simulink library "vmc"  (R2021b)
settings: Solver=VariableStepAuto  StartTime=0.0  StopTime=10.0  RelTol=1e-3
undefined symbols (not defined in the file): AVMC_ACCDeltaTqGradeGn_X_deg, AVMC_ACCDeltaTqIGain4OVRD_X_kph, AVMC_ACCDeltaTqIGain4OVRD_Y_mps2, AVMC_ACCDeltaTqIGain_X_kph, AVMC_ACCDeltaTqIGain_Y_mps2, AVMC_ACCDeltaTqPGain_X_kph, AVMC_ACCDeltaTqPGain_Y_kph, AVMC_ACCGradeofst_X_G, AVMC_ACCGradeofst_Y_pct, AVMC_ACCLoSpdTqLoLim4JP_X_kph, AVMC_ACCLoSpdTqLoLim4JP_Y_deg, AVMC_ACCLoSpdTqLowerLim_X_kph, AVMC_ACCLoSpdTqLowerLim_Y_deg, AVMC_ACCReqAccelGain_X_mps2, AVMC_ACCReqAccelGain_Y_enum, AVMC_ADSPosGFBDeltaTq_X_kph, AVMC_ADSPosGFBDeltaTq_Y_mps2, AVMC_AggressJerkPCT4AT_X_kph, AVMC_AggressJerkPCT_X_kph, AVMC_AggressLimitPCT4AT_X_kph, AVMC_AggressLimitPCT_X_kph, AVMC_DECGradeofst_X_G, AVMC_DECGradeofst_Y_pct, AVMC_DISCDeltaTqIGain_X_kph, AVMC_DISCDeltaTqIGain_Y_mps2, AVMC_DISCDeltaTqPGain_X_kph, AVMC_DISCDeltaTqPGain_Y_kph, AVMC_EPSForceSelect_X_enum, AVMC_EPSForceSelect_Y_enum, AVMC_EPSForceSelectD21_X_enum, AVMC_EPSForceSelectD21_Y_enum, AVMC_ESCRegenOut_X_kph, AVMC_ESCRegenOut_Y_Deg, AVMC_ESCRegenOutEnSpd_X_Deg, AVMC_EstPitchSlopeTs_X_kph, AVMC_GradeCompFlt_X_kph, AVMC_GyroYBandLo_X_Gps, AVMC_HoldResTq_X_kph, AVMC_ISOAccLimit_X_mps, AVMC_ISODecLimit_X_mps, AVMC_ISOJerk_X_mps, AVMC_LatESCRegenOut_X_kph, AVMC_LatESCRegenOut_Y_Deg, AVMC_LongAccDeadZone_X_kph, AVMC_LongAccFiltTsforP2_X_Gps, AVMC_MCPresBaseTq_X_bar, AVMC_MSAPedalOvrd_X_kph, AVMC_MSASpdBand_X_kph, AVMC_MSATqDownEndTq_X_kph, AVMC_MSATqDownTime_X_kph, AVMC_NegZCHoldTq_X_kph, AVMC_OPDDisSlideRate_X_Deg, AVMC_OVRD2ActSR2FCMCMD_X_mps2, AVMC_PedalTqRWhlRatio_X_Nm, AVMC_PedalTqRWhlRatio_Y_gps, AVMC_PedalTqRWhlSlipGain_X_rat, AVMC_PedalTqRWhlSlipGain_Y_kph, AVMC_PedalTqRWhSTRGGain_X_deg, AVMC_PedalTqRWhSTRGGain_Y_kph, AVMC_PosZCHoldTq_X_kph ... (+593)
libraries: hcu_lib x143, simulink x96, tqr x4, $bdroot x1, simulink_extras x1
(part 16 of 17)

== system vmc/VMC/VMC/Slide Rate  Calculation/4Wheel Calculation/RR Wheel ==
  VVMC_4WheelLongAcc_Gps : Inport
  task_time_s : Inport  Port=2
  VINP_RRRawWhlSpeed_kph : Inport  Port=3
  VTQD_GearActualPosn_enum : Inport  Port=4
  AND4 : Logic  Inputs=3  AllPortsSameDT=off  OutDataTypeStr=boolean
  Abs3 : Abs
  Add : Sum
  Add{3,8,15..16} (4 alike) : Sum  Inputs=+-
  Constant1 : Constant  Value=GRAVITY_G
  Constant11 : Constant  Value=KPH2MPS
  Constant14 : Constant  Value=ONE_PERCENT
  Constant15 : Constant  Value=KVMC_RawWhlSpeedDeadZone_kph
  Constant16 : Constant  Value=ZERO_FLOAT
  Constant17 : Constant  Value=KVMC_RawWhlSpeedDeadZone_kph
  Constant18 : Constant  Value=ONE_FLOAT
  Constant2 : Constant  Value=MPS2KPH
  Constant33 : Constant  Value=KPH2MPS
  Constant34 : Constant  Value=GRAVITY_G
  Constant35 : Constant  Value=KVMC_WhlSpdCalAccTs_c
  Constant42 : Constant  Value=KVMC_WheelSkidAccDev_Gps
  Constant43 : Constant  Value=KVMC_SkidRecVehSpdDev_kph
  Constant44 : Constant  Value=KPH2MPS
  Constant46 : Constant  Value=ENUM_GEARACTUALPOSN_D
  Constant47 : Constant  Value=ENUM_GEARACTUALPOSN_R
  Constant48 : Constant  Value=KVMC_PreVehSpdCalSW_flg
  Constant49 : Constant  Value=KVMC_RRWhlSkidReset_flg
  Constant5 : Constant  Value=KVMC_4WheelEnSkidDetSpd_kph
  Delay{,4..5,12..13,17} (6 alike) : Delay  DelayLength=1
  Divide3 : Product  Inputs=*//
  Divide7 : Product  Inputs=**//
  Equal : RelationalOperator  Operator===  OutDataTypeStr=boolean  RndMeth=Simplest
  Equal1 : RelationalOperator  Operator===  OutDataTypeStr=boolean  RndMeth=Simplest
  FirstOrderFilter3 : hcu_lib/Basic_Blocks/FirstOrderFilter
  OR : Logic  Operator=OR  AllPortsSameDT=off  OutDataTypeStr=boolean
  OR1 : Logic  Operator=OR  AllPortsSameDT=off  OutDataTypeStr=boolean
  OR2 : Logic  Operator=OR  AllPortsSameDT=off  OutDataTypeStr=boolean
  Product : Product
  Product1 : Product  Inputs=3
  Product2 : Product
  Product3 : Product
  Relational Operator14 : RelationalOperator  Operator=>  OutDataTypeStr=boolean  RndMeth=Simplest
  Relational Operator{2,5..6,15} (4 alike) : RelationalOperator  Operator=<=  OutDataTypeStr=boolean  RndMeth=Simplest
  SR_Latch3 : hcu_lib/Basic_Blocks/SR_Latch
  Saturation : Saturate  UpperLimit=KVMC_PredVehSpdLimit_mps  LowerLimit=ZERO_FLOAT
  Switch{,5..6,10} (4 alike) : Switch  Criteria=u2 > Threshold
  VVMC_RRPreVehSpd_kph : Outport
  VVMC_RRWhlSkid_flg : Outport  Port=2
  VVMC_RR4WhlSpdSlideRate_pct : Outport  Port=3
  wires:
  OR2/1 -> SR_Latch3/2  "VVMC_RRWhlSkidReset_flg"
  AND4/1 -> OR2/2
  Relational Operator2/1 -> OR2/1
  [VINP_RRRawWhlSpeed_kph] -> Relational Operator2/1
  Constant5/1 -> Relational Operator2/2
  [VVMC_RR4WhlSpdSlideRate_pct] -> VVMC_RR4WhlSpdSlideRate_pct/1
  [VVMC_RRWhlSkid_flg] -> VVMC_RRWhlSkid_flg/1
  [VVMC_RRPreVehSpd_kph] -> VVMC_RRPreVehSpd_kph/1
  VINP_RRRawWhlSpeed_kph/1 -> [VINP_RRRawWhlSpeed_kph]
  task_time_s/1 -> [task_time_s]
  VTQD_GearActualPosn_enum/1 -> [VTQD_GearActualPosn_enum]
  VVMC_4WheelLongAcc_Gps/1 -> [VVMC_4WheelLongAcc_Gps]
  [VVMC_RRPreVehSpd_kph] -> Switch5/3
  [VVMC_RRPreVehSpd_kph] -> Relational Operator5/1
  [VVMC_RRPreVehSpd_kph] -> Add3/2
  [VVMC_RRPreVehSpd_kph] -> Delay12/1
  [VINP_RRRawWhlSpeed_kph] -> Delay13/1
  [VINP_RRRawWhlSpeed_kph] -> Delay/1
  [VVMC_RRWhlSkid_flg] -> OR1/1
  OR/1 -> Switch10/2
  Product/1 -> Switch/3
  Delay5/1 -> Product3/1
  Saturation/1 -> Add/2
  Product1/1 -> Add/1  "VVMC_RRDeltaVehSpd_mps"
  Constant46/1 -> Equal/2
  OR1/1 -> Switch/2
  Constant2/1 -> Product2/2
  Constant48/1 -> OR1/2
  [VTQD_GearActualPosn_enum] -> Equal1/1
  Equal1/1 -> OR/2
  Constant47/1 -> Equal1/2
  Delay/1 -> Product/1
  [VVMC_RRPreVehSpd_kph] -> Delay5/1
  Switch/1 -> Saturation/1  "VVMC_RRLastPreVehSpd_mps"
  [task_time_s] -> Product1/3
  Constant44/1 -> Product3/2
  Constant11/1 -> Product/2
  [VVMC_4WheelLongAcc_Gps] -> Product1/1
  Product2/1 -> Switch10/1
  Equal/1 -> OR/1
  Add/1 -> Product2/1  "VVMC_RRCalPreVehSpd_mps"
  [VTQD_GearActualPosn_enum] -> Equal/1
  [VINP_RRRawWhlSpeed_kph] -> Switch10/3
  Switch10/1 -> [VVMC_RRPreVehSpd_kph]  "VVMC_RRPreVehSpd_kph"
  Constant1/1 -> Product1/2
  Product3/1 -> Switch/1
  Add3/1 -> Divide3/1
  [VINP_RRRawWhlSpeed_kph] -> Add3/1
  Constant17/1 -> Relational Operator5/2
  Constant16/1 -> Switch6/1
  Constant15/1 -> Relational Operator6/2
  Relational Operator5/1 -> Switch5/2
  [VINP_RRRawWhlSpeed_kph] -> Relational Operator6/1
  Relational Operator6/1 -> Switch6/2
  Constant18/1 -> Switch5/1
  Switch6/1 -> [VVMC_RR4WhlSpdSlideRate_pct]  "VVMC_RR4WhlSpdSlideRate_pct"
  Divide3/1 -> Switch6/3  "VVMC_RRCal4WhlSpdSlideRate_pct"
  Switch5/1 -> Divide3/3
  Constant14/1 -> Divide3/2
  Constant35/1 -> FirstOrderFilter3/3
  [VVMC_RRWhlCalAcc_Gps] -> Add16/1
  SR_Latch3/1 -> [VVMC_RRWhlSkid_flg]  "VVMC_RRWhlSkid_flg"
  Abs3/1 -> Relational Operator15/1
  Constant34/1 -> Divide7/4
  Constant33/1 -> Divide7/2
  Delay13/1 -> Add15/2
  Constant43/1 -> Relational Operator15/2
  Delay12/1 -> Add15/1
  Add16/1 -> Relational Operator14/1
  [VVMC_RRWhlSkid_flg] -> Delay17/1
  Delay17/1 -> AND4/2
  Delay4/1 -> Add8/2
  Relational Operator15/1 -> AND4/1
  Divide7/1 -> FirstOrderFilter3/1
  FirstOrderFilter3/1 -> [VVMC_RRWhlCalAcc_Gps]  "VVMC_RRWhlCalAcc_Gps"
  Constant42/1 -> Relational Operator14/2
  [VINP_RRRawWhlSpeed_kph] -> Delay4/1
  [task_time_s] -> FirstOrderFilter3/2
  [VVMC_4WheelLongAcc_Gps] -> Add16/2
  Relational Operator14/1 -> SR_Latch3/1
  Add15/1 -> Abs3/1
  [task_time_s] -> Divide7/3
  Add8/1 -> Divide7/1
  Constant49/1 -> AND4/3
  [VINP_RRRawWhlSpeed_kph] -> Add8/1

== stateflow chart vmc/VMC/VMC/IMU/IMU sensing result /RollingAverage3 ==
  state RollingAverage
    (default) -> (junction 2) : {VVMC_RollAveCount_enum = ONE_INT}
    RollingAverage -> (junction 2)
    (junction 2) -> (junction 3) : {VVMC_RollAve_raw32 = ZERO_FLOAT}
    (junction 3) -> (junction 100) [order 1] : [VVMC_RollAveCount_enum < KVMC_RollAveLevel_enum]
    (junction 3) -> (junction 37) [order 2]
    (junction 100) -> (junction 5) : {% Memory
        |  VVMC_Memory_raw32[VVMC_RollAveCount_enum] = VINP_INPData_raw32;
        |
        |  % Memory Shift Counter
        |  VVMC_ShiftCount_enum = ONE_INT}
    (junction 5) -> (junction 7) [order 2]
    (junction 5) -> (junction 6) [order 1] : [VVMC_ShiftCount_enum <= VVMC_RollAveCount_enum]
    (junction 7) -> (junction 8) : {% Rolling Average
        |  VVMC_RollAve_raw32 = VVMC_RollAve_raw32 / VVMC_RollAveCount_enum;
        |
        |  % Rolling Average Counter
        |  VVMC_RollAveCount_enum++}
    (junction 35) -> (junction 5) : {VVMC_ShiftCount_enum++}
    (junction 6) -> (junction 36) : {% Rolling Average Sum
        |  VVMC_RollAve_raw32 = VVMC_RollAve_raw32 + VVMC_Memory_raw32[VVMC_ShiftCount_enum];
        |  }
    (junction 36) -> (junction 35)
    (junction 37) -> (junction 76) [order 1] : [VVMC_RollAveCount_enum == KVMC_RollAveLevel_enum]
    (junction 76) -> (junction 47)
    (junction 37) -> (junction 60) [order 2]
    (junction 78) -> (junction 76)
    (junction 47) -> (junction 30) : {% Memory
        |  VVMC_Memory_raw32[VVMC_RollAveCount_enum] = VINP_INPData_raw32;
        |
        |  % Memory Shift Counter
        |  VVMC_ShiftCount_enum = ONE_INT;
        | }
    (junction 60) -> (junction 62) [order 1] : [VVMC_RollAveCount_enum > KVMC_RollAveLevel_enum]
    (junction 60) -> (junction 39) [order 2]
    (junction 62) -> (junction 66) : {VVMC_MemoryShiftCount_enum = ONE_INT}
    (junction 30) -> (junction 48) [order 2]
    (junction 30) -> (junction 22) [order 1] : [VVMC_ShiftCount_enum <= VVMC_RollAveCount_enum]
    (junction 48) -> (junction 45) : {% Rolling Average
        |  VVMC_RollAve_raw32 = VVMC_RollAve_raw32 / VVMC_RollAveCount_enum;
        |
        |  % Memory Shift Counter
        |  VVMC_ShiftCount_enum = ONE_INT}
    (junction 14) -> (junction 30) : {VVMC_ShiftCount_enum++}
    (junction 22) -> (junction 25) : {% Rolling Average Sum
        |  VVMC_RollAve_raw32 = VVMC_RollAve_raw32 + VVMC_Memory_raw32[VVMC_ShiftCount_enum]}
    (junction 66) -> (junction 82) [order 2]
    (junction 66) -> (junction 69) [order 1] : [VVMC_MemoryShiftCount_enum < VVMC_RollAveCount_enum]
    (junction 82) -> (junction 80) : {VVMC_RollAveCount_enum = KVMC_RollAveLevel_enum}
    (junction 73) -> (junction 66) : {VVMC_MemoryShiftCount_enum++}
    (junction 69) -> (junction 71) : {VVMC_Memory_raw32[VVMC_MemoryShiftCount_enum] =...
        |  VVMC_Memory_raw32[VVMC_RollAveCount_enum - KVMC_RollAveLevel_enum + VVMC_MemoryShiftCount_enum]}
    (junction 25) -> (junction 14)
    (junction 71) -> (junction 73)
    (junction 80) -> (junction 78)
    (junction 45) -> (junction 39) [order 2]
    (junction 45) -> (junction 15) [order 1] : [VVMC_ShiftCount_enum < VVMC_RollAveCount_enum]
    (junction 41) -> (junction 45) : { VVMC_ShiftCount_enum++}
    (junction 15) -> (junction 38) : {% Gy Memory Shift
        |  VVMC_Memory_raw32[VVMC_ShiftCount_enum] = VVMC_Memory_raw32[VVMC_ShiftCount_enum + ONE_INT]}
    (junction 38) -> (junction 41)
  data: KVMC_RollAveLevel_enum input uint8; VVMC_ShiftCount_enum local uint8; VVMC_RollAveCount_enum local uint8; VVMC_Memory_raw32 local single size=256; ZERO_FLOAT input single; ONE_INT input uint8; VVMC_RollAve_raw32 output single; VINP_INPData_raw32 input single; VVMC_MemoryShiftCount_enum local uint8

== stateflow chart vmc/VMC/VMC/IMU/IMU sensing result /RollingAverage4 ==
  state RollingAverage
    (default) -> (junction 2) : {VVMC_RollAveCount_enum = ONE_INT}
    RollingAverage -> (junction 2)
    (junction 2) -> (junction 3) : {VVMC_RollAve_raw32 = ZERO_FLOAT}
    (junction 3) -> (junction 100) [order 1] : [VVMC_RollAveCount_enum < KVMC_RollAveLevel_enum]
    (junction 3) -> (junction 37) [order 2]
    (junction 100) -> (junction 5) : {% Memory
        |  VVMC_Memory_raw32[VVMC_RollAveCount_enum] = VINP_INPData_raw32;
        |
        |  % Memory Shift Counter
        |  VVMC_ShiftCount_enum = ONE_INT}
    (junction 5) -> (junction 7) [order 2]
    (junction 5) -> (junction 6) [order 1] : [VVMC_ShiftCount_enum <= VVMC_RollAveCount_enum]
    (junction 7) -> (junction 8) : {% Rolling Average
        |  VVMC_RollAve_raw32 = VVMC_RollAve_raw32 / VVMC_RollAveCount_enum;
        |
        |  % Rolling Average Counter
        |  VVMC_RollAveCount_enum++}
    (junction 35) -> (junction 5) : {VVMC_ShiftCount_enum++}
    (junction 6) -> (junction 36) : {% Rolling Average Sum
        |  VVMC_RollAve_raw32 = VVMC_RollAve_raw32 + VVMC_Memory_raw32[VVMC_ShiftCount_enum];
        |  }
    (junction 36) -> (junction 35)
    (junction 37) -> (junction 76) [order 1] : [VVMC_RollAveCount_enum == KVMC_RollAveLevel_enum]
    (junction 76) -> (junction 47)
    (junction 37) -> (junction 60) [order 2]
    (junction 78) -> (junction 76)
    (junction 47) -> (junction 30) : {% Memory
        |  VVMC_Memory_raw32[VVMC_RollAveCount_enum] = VINP_INPData_raw32;
        |
        |  % Memory Shift Counter
        |  VVMC_ShiftCount_enum = ONE_INT;
        | }
    (junction 60) -> (junction 62) [order 1] : [VVMC_RollAveCount_enum > KVMC_RollAveLevel_enum]
    (junction 60) -> (junction 39) [order 2]
    (junction 62) -> (junction 66) : {VVMC_MemoryShiftCount_enum = ONE_INT}
    (junction 30) -> (junction 48) [order 2]
    (junction 30) -> (junction 22) [order 1] : [VVMC_ShiftCount_enum <= VVMC_RollAveCount_enum]
    (junction 48) -> (junction 45) : {% Rolling Average
        |  VVMC_RollAve_raw32 = VVMC_RollAve_raw32 / VVMC_RollAveCount_enum;
        |
        |  % Memory Shift Counter
        |  VVMC_ShiftCount_enum = ONE_INT}
    (junction 14) -> (junction 30) : {VVMC_ShiftCount_enum++}
    (junction 22) -> (junction 25) : {% Rolling Average Sum
        |  VVMC_RollAve_raw32 = VVMC_RollAve_raw32 + VVMC_Memory_raw32[VVMC_ShiftCount_enum]}
    (junction 66) -> (junction 82) [order 2]
    (junction 66) -> (junction 69) [order 1] : [VVMC_MemoryShiftCount_enum < VVMC_RollAveCount_enum]
    (junction 82) -> (junction 80) : {VVMC_RollAveCount_enum = KVMC_RollAveLevel_enum}
    (junction 73) -> (junction 66) : {VVMC_MemoryShiftCount_enum++}
    (junction 69) -> (junction 71) : {VVMC_Memory_raw32[VVMC_MemoryShiftCount_enum] =...
        |  VVMC_Memory_raw32[VVMC_RollAveCount_enum - KVMC_RollAveLevel_enum + VVMC_MemoryShiftCount_enum]}
    (junction 25) -> (junction 14)
    (junction 71) -> (junction 73)
    (junction 80) -> (junction 78)
    (junction 45) -> (junction 39) [order 2]
    (junction 45) -> (junction 15) [order 1] : [VVMC_ShiftCount_enum < VVMC_RollAveCount_enum]
    (junction 41) -> (junction 45) : { VVMC_ShiftCount_enum++}
    (junction 15) -> (junction 38) : {% Gy Memory Shift
        |  VVMC_Memory_raw32[VVMC_ShiftCount_enum] = VVMC_Memory_raw32[VVMC_ShiftCount_enum + ONE_INT]}
    (junction 38) -> (junction 41)
  data: KVMC_RollAveLevel_enum input uint8; VVMC_ShiftCount_enum local uint8; VVMC_RollAveCount_enum local uint8; VVMC_Memory_raw32 local single size=256; ZERO_FLOAT input single; ONE_INT input uint8; VVMC_RollAve_raw32 output single; VINP_INPData_raw32 input single; VVMC_MemoryShiftCount_enum local uint8

== stateflow chart vmc/VMC/VMC/IMU/IMU sensing result /RollingAverage5 ==
  state RollingAverage
    (default) -> (junction 2) : {VVMC_RollAveCount_enum = ONE_INT}
    RollingAverage -> (junction 2)
    (junction 2) -> (junction 3) : {VVMC_RollAve_raw32 = ZERO_FLOAT}
    (junction 3) -> (junction 100) [order 1] : [VVMC_RollAveCount_enum < KVMC_RollAveLevel_enum]
    (junction 3) -> (junction 37) [order 2]
    (junction 100) -> (junction 5) : {% Memory
        |  VVMC_Memory_raw32[VVMC_RollAveCount_enum] = VINP_INPData_raw32;
        |
        |  % Memory Shift Counter
        |  VVMC_ShiftCount_enum = ONE_INT}
    (junction 5) -> (junction 7) [order 2]
    (junction 5) -> (junction 6) [order 1] : [VVMC_ShiftCount_enum <= VVMC_RollAveCount_enum]
    (junction 7) -> (junction 8) : {% Rolling Average
        |  VVMC_RollAve_raw32 = VVMC_RollAve_raw32 / VVMC_RollAveCount_enum;
        |
        |  % Rolling Average Counter
        |  VVMC_RollAveCount_enum++}
    (junction 35) -> (junction 5) : {VVMC_ShiftCount_enum++}
    (junction 6) -> (junction 36) : {% Rolling Average Sum
        |  VVMC_RollAve_raw32 = VVMC_RollAve_raw32 + VVMC_Memory_raw32[VVMC_ShiftCount_enum];
        |  }
    (junction 36) -> (junction 35)
    (junction 37) -> (junction 76) [order 1] : [VVMC_RollAveCount_enum == KVMC_RollAveLevel_enum]
    (junction 76) -> (junction 47)
    (junction 37) -> (junction 60) [order 2]
    (junction 78) -> (junction 76)
    (junction 47) -> (junction 30) : {% Memory
        |  VVMC_Memory_raw32[VVMC_RollAveCount_enum] = VINP_INPData_raw32;
        |
        |  % Memory Shift Counter
        |  VVMC_ShiftCount_enum = ONE_INT;
        | }
    (junction 60) -> (junction 62) [order 1] : [VVMC_RollAveCount_enum > KVMC_RollAveLevel_enum]
    (junction 60) -> (junction 39) [order 2]
    (junction 62) -> (junction 66) : {VVMC_MemoryShiftCount_enum = ONE_INT}
    (junction 30) -> (junction 48) [order 2]
    (junction 30) -> (junction 22) [order 1] : [VVMC_ShiftCount_enum <= VVMC_RollAveCount_enum]
    (junction 48) -> (junction 45) : {% Rolling Average
        |  VVMC_RollAve_raw32 = VVMC_RollAve_raw32 / VVMC_RollAveCount_enum;
        |
        |  % Memory Shift Counter
        |  VVMC_ShiftCount_enum = ONE_INT}
    (junction 14) -> (junction 30) : {VVMC_ShiftCount_enum++}
    (junction 22) -> (junction 25) : {% Rolling Average Sum
        |  VVMC_RollAve_raw32 = VVMC_RollAve_raw32 + VVMC_Memory_raw32[VVMC_ShiftCount_enum]}
    (junction 66) -> (junction 82) [order 2]
    (junction 66) -> (junction 69) [order 1] : [VVMC_MemoryShiftCount_enum < VVMC_RollAveCount_enum]
    (junction 82) -> (junction 80) : {VVMC_RollAveCount_enum = KVMC_RollAveLevel_enum}
    (junction 73) -> (junction 66) : {VVMC_MemoryShiftCount_enum++}
    (junction 69) -> (junction 71) : {VVMC_Memory_raw32[VVMC_MemoryShiftCount_enum] =...
        |  VVMC_Memory_raw32[VVMC_RollAveCount_enum - KVMC_RollAveLevel_enum + VVMC_MemoryShiftCount_enum]}
    (junction 25) -> (junction 14)
    (junction 71) -> (junction 73)
    (junction 80) -> (junction 78)
    (junction 45) -> (junction 39) [order 2]
    (junction 45) -> (junction 15) [order 1] : [VVMC_ShiftCount_enum < VVMC_RollAveCount_enum]
    (junction 41) -> (junction 45) : { VVMC_ShiftCount_enum++}
    (junction 15) -> (junction 38) : {% Gy Memory Shift
        |  VVMC_Memory_raw32[VVMC_ShiftCount_enum] = VVMC_Memory_raw32[VVMC_ShiftCount_enum + ONE_INT]}
    (junction 38) -> (junction 41)
  data: KVMC_RollAveLevel_enum input uint8; VVMC_ShiftCount_enum local uint8; VVMC_RollAveCount_enum local uint8; VVMC_Memory_raw32 local single size=256; ZERO_FLOAT input single; ONE_INT input uint8; VVMC_RollAve_raw32 output single; VINP_INPData_raw32 input single; VVMC_MemoryShiftCount_enum local uint8

== stateflow chart vmc/VMC/VMC/MSA function/MSAActivationHandshake/Chart ==
  state MSA_Handshaking
    (default) -> (junction 391) : {VVMC_IntMSACtrlSta_enum = 0;
        |  VVMC_IntMSASpdWar_flg = 0;
        |  VVMC_WaitResetSpdLoop_flg = 0;}
    MSA_Handshaking -> (junction 391) [order 4] : {VVMC_WaitResetSpdLoop_flg = 0;
        |  VVMC_CheckMeterSpdLoop_flg = 0;
        |  VVMC_CheckCmdLoop_flg = 0}
    (junction 391) -> (junction 463) [order 1] : [(VTQD_SpdCtrlMode_enum == 3 ||...
        |  VTQD_SpdCtrlMode_enum == 4) && ...
        |  VVMC_VMCMSACtrlAvail_flg &&... %241026
        |  VTQD_GearActualPosn_enum == ENUM_GEARACTUALPOSN_D]
        | %add20230706
    (junction 463) -> (junction 392) [order 1] : [VTQD_ExternalTqAllow_flg]
    (junction 391) -> (junction 467) [order 2] : {VVMC_IntMSACtrlSta_enum = 0;}
        | %Phase2 VVMC_MSAActive_flg = 0;}
        | %add20230706
    (junction 463) -> (junction 468) [order 2] : {VVMC_IntMSACtrlSta_enum = 5;}
        | %Phase2  VVMC_MSAActive_flg = 0;}
        | %add20230706
    (junction 392) -> (junction 389) : {VVMC_IntMSACtrlSta_enum = 1;}
    MSA_Handshaking -> (junction 389) [order 3] : [VVMC_WaitResetSpdLoop_flg && VTQD_ExternalTqAllow_flg]
        | {VVMC_WaitResetSpdLoop_flg = 0;} %add20230705
    (junction 389) -> (junction 464) [order 1] : [VVMC_DetectSWCSet_flg &&... %241022
        |  VVMC_FeatSetSpdFinal_raw32 > ONE_FLOAT]
    (junction 389) -> (junction 469) [order 2]
    (junction 464) -> (junction 330)
    MSA_Handshaking -> (junction 330) [order 1] : [VVMC_CheckMeterSpdLoop_flg && VTQD_ExternalTqAllow_flg]
        | {VVMC_CheckMeterSpdLoop_flg = 0;}
        | %Phase2 add
    (junction 330) -> (junction 332) [order 1] : [VVMC_FeatSetSpdFinal_raw32 >= KVMC_MSAActiveMetSpdLo_kph &&...
        |  VVMC_FeatSetSpdFinal_raw32 <=  KVMC_MSAActiveMetSpdHi_kph]
    (junction 330) -> (junction 338) [order 2] : {VVMC_IntMSASpdWar_flg = 0;}
    (junction 332) -> (junction 335) : {VVMC_IntMSACtrlSta_enum = 2;}
        | %Phase2 VVMC_MSAActive_flg = 1;}
    (junction 338) -> (junction 339) [order 1] : [VVMC_FeatSetSpdFinal_raw32 > KVMC_MSAActiveMetSpdHi_kph]
    (junction 335) -> (junction 336) [order 1] : [(VVMC_MeterIndSpeed_raw32 - VVMC_FeatSetSpdFinal_raw32)...
        | >= KVMC_CCMSASpdWar_raw32]
    (junction 338) -> (junction 334) [order 2] : {VVMC_IntMSACtrlSta_enum = 3;}
    (junction 339) -> (junction 333) : {VVMC_IntMSACtrlSta_enum = 4;}
    (junction 335) -> (junction 346) [order 2] : {VVMC_IntMSASpdWar_flg = 0;}
    (junction 336) -> (junction 345) : {VVMC_IntMSASpdWar_flg = 1;}
    (junction 334) -> (junction 333)
    (junction 333) -> (junction 337) : {VVMC_WaitResetSpdLoop_flg = 1;}
    (junction 346) -> (junction 345)
    (junction 345) -> (junction 342) [order 1] : [(VTQD_SpdCtrlMode_enum != 3 && VTQD_SpdCtrlMode_enum != 4) ||...
        |   VVMC_DetectSWCCANCEL_flg == 1||...
        |  !VTQD_ExternalTqAllow_flg] %Phase2 add20230815
        | %add20230706
    (junction 345) -> (junction 471) [order 2]
    (junction 342) -> (junction 348) : {VVMC_IntMSASpdWar_flg = 0;}
    (junction 471) -> (junction 472) [order 1] : [VVMC_MSAOvrdAllow_flg == 1]
    (junction 471) -> (junction 474) [order 2] : {VVMC_IntMSACtrlSta_enum = 2;}
    (junction 472) -> (junction 473) : {VVMC_IntMSACtrlSta_enum = 7;}
    (junction 474) -> (junction 473)
    (junction 473) -> (junction 347) : {VVMC_CheckMeterSpdLoop_flg = 1;}
    (junction 348) -> (junction 343) [order 1] : [!VTQD_ExternalTqAllow_flg] %Phase2 add20230815
    (junction 348) -> (junction 360) [order 2]
    (junction 343) -> (junction 344) : %Phase2 add20230815
        | {VVMC_IntMSACtrlSta_enum = 5;}
        | %Back to outer first loop.
    MSA_Handshaking -> (junction 360) [order 2] : [VVMC_CheckCmdLoop_flg && VTQD_ExternalTqAllow_flg]
        | {VVMC_CheckCmdLoop_flg = 0;} %Phase2 add 20231003
    (junction 360) -> (junction 350) [order 1] : [(VTQD_SpdCtrlMode_enum != 3 && VTQD_SpdCtrlMode_enum != 4)] %241018 %Phase2 add
    (junction 360) -> (junction 353) [order 2] : %Phase2 {VVMC_MSAActive_flg = 0;
        | {VVMC_IntMSACtrlSta_enum = 1;}
    (junction 350) -> (junction 373) : %Phase2 {VVMC_MSAActive_flg = 0;
        | {VVMC_IntMSACtrlSta_enum = 0;}
        |  %Back to outer first loop.
    (junction 353) -> (junction 354) [order 1] : [VVMC_DetectSWCRes_flg == 1 ||...
        |  VVMC_DetectSWCSet_flg == 1]
        | %Phase2 add
    (junction 353) -> (junction 370) [order 2] : {VVMC_CheckCmdLoop_flg = 1}
        | %Phase2 Modify 20231003
    (junction 354) -> (junction 349) : {VVMC_CheckMeterSpdLoop_flg = 1}
        | %Phase2 add
  MSA_Handshaking -> MSA_Handshaking [order 1] : [!VTQD_ExternalTqAllow_flg || VTQD_GearActualPosn_enum ~= ENUM_GEARACTUALPOSN_D ||...
      |  (VTQD_SpdCtrlMode_enum != 3 && VTQD_SpdCtrlMode_enum != 4) || !VVMC_VMCMSACtrlAvail_flg] %241018
      | %add20240906
  data: VTQD_SpdCtrlMode_enum input uint8; VVMC_IntMSACtrlSta_enum output uint8; VVMC_IntMSASpdWar_flg output boolean; VTQD_ExternalTqAllow_flg input boolean; KVMC_MSAActiveMetSpdHi_kph input single; VVMC_MeterIndSpeed_raw32 input single; KVMC_MSAActiveMetSpdLo_kph input single; VVMC_FeatSetSpdFinal_raw32 input single; KVMC_CCMSASpdWar_raw32 input single; VVMC_DetectSWCCANCEL_flg input boolean; VVMC_MSAOvrdAllow_flg input; VVMC_CheckMeterSpdLoop_flg local boolean; VVMC_WaitResetSpdLoop_flg local boolean; VVMC_DetectSWCRes_flg input boolean; VVMC_DetectSWCSet_flg input boolean; VVMC_CheckCmdLoop_flg local boolean; ONE_FLOAT parameter; VTQD_GearActualPosn_enum input; ENUM_GEARACTUALPOSN_D parameter; VVMC_VMCMSACtrlAvail_flg input

== stateflow chart vmc/VMC/VMC/SPD2ACC/SPD2ACC Active Determination/SPD2ACC Active Determination ==
  state SPD2ACCActiveDetermination
    (default) -> (junction 4) : {VVMC_SPD2ACCAct_flg = FALSE}
    SPD2ACCActiveDetermination -> (junction 4)
    (junction 4) -> (junction 7) [order 1] : [VVMC_FeatArbitrSta_enum == ENUM_FEATARBITRSTA_DISC ||...
        |  VVMC_FeatArbitrSta_enum == ENUM_FEATARBITRSTA_CC ||...
        |  VVMC_FeatArbitrSta_enum == ENUM_FEATARBITRSTA_MSA ||...
        |  VVMC_FeatArbitrSta_enum == ENUM_FEATARBITRSTA_ACCDISC]
    (junction 4) -> (junction 12) [order 2] : {VVMC_SPD2ACCAct_flg = FALSE}
    (junction 7) -> (junction 10) : {VVMC_SPD2ACCAct_flg = TURE}
  data: VVMC_FeatArbitrSta_enum input uint8; VVMC_SPD2ACCAct_flg output boolean; TURE input boolean; FALSE input boolean; ENUM_FEATARBITRSTA_DISC input uint8; ENUM_FEATARBITRSTA_ACCDISC input uint8; ENUM_FEATARBITRSTA_CC input; ENUM_FEATARBITRSTA_MSA input

== stateflow chart vmc/VMC/VMC/SPD2ACC/Required_Acceleration/CMDRepeat ==
  state CMDCycleTime
    (default) -> (junction 4) : {VVMC_CMDCount_enum = ZERO_INT}
    CMDCycleTime -> (junction 4)
    (junction 4) -> (junction 8) [order 1] : [VVMC_SPD2ACCAct_flg == TRUE &&...
        | (VVMC_DISCReqAccAftLim_mps2 > ZERO_FLOAT ||...
        |  VVMC_DISCReqAccAftLim_mps2 < ZERO_FLOAT)]
    (junction 8) -> (junction 13) [order 1] : [VVMC_CMDCount_enum == ZERO_INT ||...
        |  KVMC_CMDRepeatTime_enum == ZERO_INT]
    (junction 13) -> (junction 31) [order 1] : [KVMC_CMDRepeatTime_enum == ZERO_INT]
    (junction 4) -> (junction 21) [order 2] : {VVMC_DISCReqAccAftRepeat_mps2 = ZERO_FLOAT;
        |  VVMC_CMDCount_enum = ZERO_INT}
    (junction 8) -> (junction 11) [order 2]
    (junction 13) -> (junction 15) [order 2] : {VVMC_DISCReqAccAftRepeat_mps2 = VVMC_DISCReqAccAftLim_mps2;
        |  VVMC_CMDCount_enum++}
    (junction 31) -> (junction 33) : {VVMC_DISCReqAccAftRepeat_mps2 = VVMC_DISCReqAccAftLim_mps2;}
    (junction 11) -> (junction 17) [order 1] : [VVMC_CMDCount_enum < KVMC_CMDRepeatTime_enum]
    (junction 11) -> (junction 23) [order 2] : {VVMC_CMDCount_enum = ZERO_INT}
    (junction 17) -> (junction 19) : {VVMC_CMDCount_enum++}
  data: VVMC_DISCReqAccAftLim_mps2 input single; TRUE input; ZERO_FLOAT input; VVMC_CMDCount_enum local uint8; VVMC_DISCReqAccAftRepeat_mps2 output single; ZERO_INT input uint8; KVMC_CMDRepeatTime_enum input uint8; VVMC_SPD2ACCAct_flg input

== stateflow chart vmc/VMC/VMC/SPD2ACC/Required_Acceleration/ConstantSpeedControl ==
  state ConstantSpeedControl
    (default) -> (junction 2) : {SpdCtrlFlag = 0;
        |  ReqAccel = 0}
    ConstantSpeedControl -> (junction 2)
    (junction 2) -> (junction 6) [order 1] : [DeltaSpeed >= KVMC_SpdCtrlEnBand_kph && SpdCtrlFlag == 0 && ZeroDeltaSpd]
    (junction 2) -> (junction 16) [order 2]
    (junction 6) -> (junction 8) : {SpdCtrlFlag = 1;
        |  ReqAccel = MINUSONE_FLOAT * KVMC_SpdCtrlReqAccel_mps2}
    (junction 16) -> (junction 15) [order 1] : [DeltaSpeed <= MINUSONE_FLOAT * KVMC_SpdCtrlEnBand_kph && SpdCtrlFlag == 0 && ZeroDeltaSpd]
    (junction 16) -> (junction 20) [order 2]
    (junction 15) -> (junction 12) : {SpdCtrlFlag = 1;
        |  ReqAccel = KVMC_SpdCtrlReqAccel_mps2}
    (junction 20) -> (junction 18) [order 1] : [ZeroDeltaSpd && SpdCtrlFlag == 1]
    (junction 18) -> (junction 24) [order 1] : [ReqAccel > ZERO_FLOAT]
    (junction 24) -> (junction 26) [order 1] : [DeltaSpeed >= KVMC_SpdCtrlDisBand_kph]
    (junction 20) -> (junction 42) [order 2] : {SpdCtrlFlag = 0;
        |  ReqAccel = ZERO_FLOAT}
    (junction 18) -> (junction 40) [order 2]
    (junction 24) -> (junction 30) [order 2] : {SpdCtrlFlag = 1;
        |  ReqAccel = KVMC_SpdCtrlReqAccel_mps2}
    (junction 26) -> (junction 28) : {SpdCtrlFlag = 0;
        |  ReqAccel = ZERO_FLOAT}
    (junction 40) -> (junction 37) [order 1] : [ReqAccel < ZERO_FLOAT]
    (junction 37) -> (junction 33) [order 1] : [DeltaSpeed <= MINUSONE_FLOAT * KVMC_SpdCtrlDisBand_kph]
    (junction 40) -> (junction 49) [order 2]
    (junction 37) -> (junction 35) [order 2] : {SpdCtrlFlag = 1;
        |  ReqAccel = MINUSONE_FLOAT * KVMC_SpdCtrlReqAccel_mps2}
    (junction 33) -> (junction 38) : {SpdCtrlFlag = 0;
        |  ReqAccel = ZERO_FLOAT}
  data: ZeroDeltaSpd input; DeltaSpeed input single; SpdCtrlFlag local boolean; ReqAccel output single; KVMC_SpdCtrlEnBand_kph input single; KVMC_SpdCtrlDisBand_kph input single; MINUSONE_FLOAT input single; KVMC_SpdCtrlReqAccel_mps2 input single; ZERO_FLOAT input single

== stateflow chart vmc/VMC/VMC/SPD2ACC/Required_Acceleration/ConstantSpeedControl1 ==
  state ConstantSpeedControl
    (default) -> (junction 2) : {SpdCtrlFlag = 0;
        |  ReqAccel = 0}
    ConstantSpeedControl -> (junction 2)
    (junction 2) -> (junction 6) [order 1] : [DeltaSpeed >= KVMC_SpdCtrlEnBand_kph && SpdCtrlFlag == 0 && VVMC_ACCSpdCtrl_flg]
    (junction 2) -> (junction 16) [order 2]
    (junction 6) -> (junction 8) : {SpdCtrlFlag = 1;
        |  ReqAccel = MINUSONE_FLOAT * KVMC_SpdCtrlReqAccel_mps2}
    (junction 16) -> (junction 15) [order 1] : [DeltaSpeed <= MINUSONE_FLOAT * KVMC_SpdCtrlEnBand_kph && SpdCtrlFlag == 0 && VVMC_ACCSpdCtrl_flg]
    (junction 16) -> (junction 20) [order 2]
    (junction 15) -> (junction 12) : {SpdCtrlFlag = 1;
        |  ReqAccel = KVMC_SpdCtrlReqAccel_mps2}
    (junction 20) -> (junction 18) [order 1] : [VVMC_ACCSpdCtrl_flg && SpdCtrlFlag == 1]
    (junction 18) -> (junction 24) [order 1] : [ReqAccel > ZERO_FLOAT]
    (junction 24) -> (junction 26) [order 1] : [DeltaSpeed >= KVMC_SpdCtrlDisBand_kph]
    (junction 20) -> (junction 42) [order 2] : {SpdCtrlFlag = 0;
        |  ReqAccel = ZERO_FLOAT}
    (junction 18) -> (junction 40) [order 2]
    (junction 24) -> (junction 30) [order 2] : {SpdCtrlFlag = 1;
        |  ReqAccel = KVMC_SpdCtrlReqAccel_mps2}
    (junction 26) -> (junction 28) : {SpdCtrlFlag = 0;
        |  ReqAccel = ZERO_FLOAT}
    (junction 40) -> (junction 37) [order 1] : [ReqAccel < ZERO_FLOAT]
    (junction 37) -> (junction 33) [order 1] : [DeltaSpeed <= MINUSONE_FLOAT * KVMC_SpdCtrlDisBand_kph]
    (junction 40) -> (junction 49) [order 2]
    (junction 37) -> (junction 35) [order 2] : {SpdCtrlFlag = 1;
        |  ReqAccel = MINUSONE_FLOAT * KVMC_SpdCtrlReqAccel_mps2}
    (junction 33) -> (junction 38) : {SpdCtrlFlag = 0;
        |  ReqAccel = ZERO_FLOAT}
  data: DeltaSpeed input single; SpdCtrlFlag local boolean; ReqAccel output single; KVMC_SpdCtrlEnBand_kph input single; KVMC_SpdCtrlDisBand_kph input single; MINUSONE_FLOAT input single; KVMC_SpdCtrlReqAccel_mps2 input single; ZERO_FLOAT input single; VVMC_ACCSpdCtrl_flg input

== stateflow chart vmc/VMC/VMC/SafetyControl/LatAccRollingAverage/RollingAverage ==
  state LatAccelRollingAverage
    (default) -> (junction 2) : {VVMC_RollAveCount_enum = ONE_INT}
    LatAccelRollingAverage -> (junction 2)
    (junction 2) -> (junction 3) : {VVMC_LatAccRollAveRaw_Gps = ZERO_FLOAT}
    (junction 3) -> (junction 100) [order 1] : [VVMC_RollAveCount_enum < KVMC_LatAccRollAveLevel_enum]
    (junction 3) -> (junction 37) [order 2]
    (junction 100) -> (junction 5) : {% Memory
        |  VVMC_Memory_raw32[VVMC_RollAveCount_enum] = VINP_LatAccel_Gps;
        |
        |  % Memory Shift Counter
        |  VVMC_ShiftCount_enum = ONE_INT}
    (junction 5) -> (junction 7) [order 2]
    (junction 5) -> (junction 6) [order 1] : [VVMC_ShiftCount_enum <= VVMC_RollAveCount_enum]
    (junction 7) -> (junction 8) : {% Rolling Average
        |  VVMC_LatAccRollAveRaw_Gps = VVMC_LatAccRollAveRaw_Gps / VVMC_RollAveCount_enum;
        |
        |  % Rolling Average Counter
        |  VVMC_RollAveCount_enum++}
    (junction 35) -> (junction 5) : {VVMC_ShiftCount_enum++}
    (junction 6) -> (junction 36) : {% Rolling Average Sum
        |  VVMC_LatAccRollAveRaw_Gps = VVMC_LatAccRollAveRaw_Gps + VVMC_Memory_raw32[VVMC_ShiftCount_enum];
        |  }
    (junction 36) -> (junction 35)
    (junction 37) -> (junction 76) [order 1] : [VVMC_RollAveCount_enum == KVMC_LatAccRollAveLevel_enum]
    (junction 76) -> (junction 47)
    (junction 37) -> (junction 60) [order 2]
    (junction 78) -> (junction 76)
    (junction 47) -> (junction 30) : {% Memory
        |  VVMC_Memory_raw32[VVMC_RollAveCount_enum] = VINP_LatAccel_Gps;
        |
        |  % Memory Shift Counter
        |  VVMC_ShiftCount_enum = ONE_INT;
        | }
    (junction 60) -> (junction 62) [order 1] : [VVMC_RollAveCount_enum > KVMC_LatAccRollAveLevel_enum]
    (junction 60) -> (junction 39) [order 2]
    (junction 62) -> (junction 66) : {VVMC_MemoryShiftCount_enum = ONE_INT}
    (junction 30) -> (junction 48) [order 2]
    (junction 30) -> (junction 22) [order 1] : [VVMC_ShiftCount_enum <= VVMC_RollAveCount_enum]
    (junction 48) -> (junction 45) : {% Rolling Average
        |  VVMC_LatAccRollAveRaw_Gps = VVMC_LatAccRollAveRaw_Gps / VVMC_RollAveCount_enum;
        |
        |  % Memory Shift Counter
        |  VVMC_ShiftCount_enum = ONE_INT}
    (junction 14) -> (junction 30) : {VVMC_ShiftCount_enum++}
    (junction 22) -> (junction 25) : {% Rolling Average Sum
        |  VVMC_LatAccRollAveRaw_Gps = VVMC_LatAccRollAveRaw_Gps + VVMC_Memory_raw32[VVMC_ShiftCount_enum]}
    (junction 66) -> (junction 82) [order 2]
    (junction 66) -> (junction 69) [order 1] : [VVMC_MemoryShiftCount_enum < VVMC_RollAveCount_enum]
    (junction 82) -> (junction 80) : {VVMC_RollAveCount_enum = KVMC_LatAccRollAveLevel_enum}
    (junction 73) -> (junction 66) : {VVMC_MemoryShiftCount_enum++}
    (junction 69) -> (junction 71) : {VVMC_Memory_raw32[VVMC_MemoryShiftCount_enum] =...
        |  VVMC_Memory_raw32[VVMC_RollAveCount_enum - KVMC_LatAccRollAveLevel_enum + VVMC_MemoryShiftCount_enum]}
    (junction 25) -> (junction 14)
    (junction 71) -> (junction 73)
    (junction 80) -> (junction 78)
    (junction 45) -> (junction 39) [order 2]
    (junction 45) -> (junction 15) [order 1] : [VVMC_ShiftCount_enum < VVMC_RollAveCount_enum]
    (junction 41) -> (junction 45) : { VVMC_ShiftCount_enum++}
    (junction 15) -> (junction 38) : {% Gy Memory Shift
        |  VVMC_Memory_raw32[VVMC_ShiftCount_enum] = VVMC_Memory_raw32[VVMC_ShiftCount_enum + ONE_INT]}
    (junction 38) -> (junction 41)
  data: KVMC_LatAccRollAveLevel_enum input uint8; VVMC_ShiftCount_enum local uint8; VVMC_RollAveCount_enum local uint8; VVMC_Memory_raw32 local single size=256; ZERO_FLOAT input single; ONE_INT input uint8; VINP_LatAccel_Gps input single; VVMC_MemoryShiftCount_enum local uint8; VVMC_LatAccRollAveRaw_Gps output single

== stateflow chart vmc/VMC/VMC/SafetyControl/SafetyControlJudgement/FrontRearSlipRatio/FrontRearSlipRatioJudgement ==
  state FrontRearSlipRatioJudgement
    (default) -> (junction 14) : {VVMC_FrontRearSlipRatioCtrl_flg = FALSE;
        |  VVMC_FrontAxleWhlSpeedAve_kph = ZERO_FLOAT;
        |  VVMC_RearAxleWhlSpeedAve_kph = ZERO_FLOAT}
    FrontRearSlipRatioJudgement -> (junction 14)
    (junction 14) -> (junction 41) [order 1] : [VINP_LFRawWhlSpeedV_flg == TRUE ||...
        |  VINP_RFRawWhlSpeedV_flg == TRUE]
    (junction 41) -> (junction 69) [order 1] : [VINP_LFRawWhlSpeedV_flg == TRUE &&...
        |  VINP_RFRawWhlSpeedV_flg == TRUE]
    (junction 14) -> (junction 54) [order 2] : {VVMC_FrontAxleWhlSpeedAve_kph =...
        | (VVMC_LFWhlSpeedRollAve_kph+VVMC_RFWhlSpeedRollAve_kph)/TWO_FLOAT}
    (junction 41) -> (junction 52) [order 2]
    (junction 69) -> (junction 47) : {VVMC_FrontRearSlipRatioCtrl_flg = FALSE}
    (junction 52) -> (junction 42) [order 1] : [VINP_LFRawWhlSpeedV_flg == TRUE]
    (junction 52) -> (junction 46) [order 2] : {VVMC_FrontAxleWhlSpeedAve_kph = VVMC_LFWhlSpeedRollAve_kph}
    (junction 42) -> (junction 49) : {VVMC_FrontAxleWhlSpeedAve_kph = VVMC_RFWhlSpeedRollAve_kph}
    (junction 46) -> (junction 54)
    (junction 49) -> (junction 46)
    (junction 54) -> (junction 92)
    (junction 92) -> (junction 85) [order 1] : [VINP_LRRawWhlSpeedV_flg == TRUE ||...
        |  VINP_RRRawWhlSpeedV_flg == TRUE]
    (junction 85) -> (junction 77) [order 1] : [VINP_LRRawWhlSpeedV_flg == TRUE &&...
        |  VINP_RRRawWhlSpeedV_flg == TRUE]
    (junction 92) -> (junction 80) [order 2] : {VVMC_RearAxleWhlSpeedAve_kph =...
        | (VVMC_LRWhlSpeedRollAve_kph+VVMC_RRWhlSpeedRollAve_kph)/TWO_FLOAT}
    (junction 85) -> (junction 89) [order 2]
    (junction 77) -> (junction 79) : {VVMC_FrontRearSlipRatioCtrl_flg = FALSE}
    (junction 89) -> (junction 84) [order 1] : [VINP_LRRawWhlSpeedV_flg == TRUE]
    (junction 89) -> (junction 82) [order 2] : {VVMC_RearAxleWhlSpeedAve_kph = VVMC_LRWhlSpeedRollAve_kph}
    (junction 84) -> (junction 78) : {VVMC_RearAxleWhlSpeedAve_kph = VVMC_RRWhlSpeedRollAve_kph}
    (junction 82) -> (junction 80)
    (junction 78) -> (junction 82)
    (junction 80) -> (junction 96)
    (junction 96) -> (junction 98) [order 1] : [abs(VVMC_RearAxleWhlSpeedAve_kph - VVMC_FrontAxleWhlSpeedAve_kph) >= KVMC_FrontRearSlipRatioTHR_kph]
    (junction 96) -> (junction 103) [order 2] : {VVMC_FrontRearSlipRatioCtrl_flg = FALSE}
    (junction 98) -> (junction 100) : {VVMC_FrontRearSlipRatioCtrl_flg = TRUE}
  data: VVMC_LFWhlSpeedRollAve_kph input single; VVMC_RFWhlSpeedRollAve_kph input single; VVMC_LRWhlSpeedRollAve_kph input single; VVMC_RRWhlSpeedRollAve_kph input single; VINP_LFRawWhlSpeedV_flg input boolean; VINP_RFRawWhlSpeedV_flg input boolean; VINP_LRRawWhlSpeedV_flg input boolean; VINP_RRRawWhlSpeedV_flg input boolean; KVMC_FrontRearSlipRatioTHR_kph input single; TRUE input boolean; VVMC_FrontRearSlipRatioCtrl_flg output boolean; FALSE input boolean; TWO_FLOAT input single; VVMC_FrontAxleWhlSpeedAve_kph local single; ZERO_FLOAT input single; VVMC_RearAxleWhlSpeedAve_kph local single

== stateflow chart vmc/VMC/VMC/SafetyControl/SafetyControlJudgement/RearWheelSlipRatio/FrontRearSlipRatioJudgement ==
  state RearWheelSlipRatioJudgement
    (default) -> (junction 14) : {VVMC_RearWhlSlipRatioCtrl_flg = FALSE}
    RearWheelSlipRatioJudgement -> (junction 14)
    (junction 14) -> (junction 85) [order 1] : [VINP_LRRawWhlSpeedV_flg == TRUE ||...
        |  VINP_RRRawWhlSpeedV_flg == TRUE]
    (junction 14) -> (junction 96) [order 2]
    (junction 85) -> (junction 105) : {VVMC_RearWhlSlipRatioCtrl_flg = FALSE}
    (junction 96) -> (junction 98) [order 1] : [abs(VVMC_LRWhlSpeedRollAve_kph - VVMC_RRWhlSpeedRollAve_kph) >= KVMC_RearWhlSlipRatioTHR_kph]
    (junction 96) -> (junction 103) [order 2] : {VVMC_RearWhlSlipRatioCtrl_flg = FALSE}
    (junction 98) -> (junction 100) : {VVMC_RearWhlSlipRatioCtrl_flg = TRUE}
  data: VVMC_LRWhlSpeedRollAve_kph input single; VVMC_RRWhlSpeedRollAve_kph input single; VINP_LRRawWhlSpeedV_flg input boolean; VINP_RRRawWhlSpeedV_flg input boolean; KVMC_RearWhlSlipRatioTHR_kph input single; TRUE input boolean; VVMC_RearWhlSlipRatioCtrl_flg output boolean; FALSE input boolean

== stateflow chart vmc/VMC/VMC/SafetyControl/SafetyControlJudgement/SingleWheelSlipRatio/SingleWheelSlipRatioJudgement ==
  state SingleWheelSlipRatioJudgement
    (default) -> (junction 14) : {VVMC_SingleWhlSlipRatioCtrl_flg = FALSE}
    SingleWheelSlipRatioJudgement -> (junction 14)
    (junction 14) -> (junction 105) [order 1] : [VINP_LFRawWhlSpeedV_flg == FALSE]
    (junction 105) -> (junction 117) [order 1] : [abs(VVMC_VehicleSpeed_kph - VVMC_LFWhlSpeedRollAve_kph) >= KVMC_SingleWhlSlipRatioTHR_kph]
    (junction 14) -> (junction 121) [order 2]
    (junction 105) -> (junction 119) [order 2]
    (junction 117) -> (junction 107) : {VVMC_SingleWhlSlipRatioCtrl_flg = TRUE}
    (junction 119) -> (junction 121)
    (junction 121) -> (junction 134)
    (junction 134) -> (junction 130) [order 1] : [VINP_RFRawWhlSpeedV_flg == FALSE]
    (junction 130) -> (junction 125) [order 1] : [abs(VVMC_VehicleSpeed_kph - VVMC_RFWhlSpeedRollAve_kph) >= KVMC_SingleWhlSlipRatioTHR_kph]
    (junction 134) -> (junction 127) [order 2]
    (junction 130) -> (junction 132) [order 2]
    (junction 125) -> (junction 131) : {VVMC_SingleWhlSlipRatioCtrl_flg = TRUE}
    (junction 132) -> (junction 127)
    (junction 127) -> (junction 143)
    (junction 143) -> (junction 149) [order 1] : [VINP_LRRawWhlSpeedV_flg == FALSE]
    (junction 149) -> (junction 144) [order 1] : [abs(VVMC_VehicleSpeed_kph - VVMC_LRWhlSpeedRollAve_kph) >= KVMC_SingleWhlSlipRatioTHR_kph]
    (junction 143) -> (junction 137) [order 2]
    (junction 149) -> (junction 146) [order 2]
    (junction 144) -> (junction 148) : {VVMC_SingleWhlSlipRatioCtrl_flg = TRUE}
    (junction 146) -> (junction 137)
    (junction 137) -> (junction 154)
    (junction 154) -> (junction 153) [order 1] : [VINP_RRRawWhlSpeedV_flg == FALSE]
    (junction 153) -> (junction 150) [order 1] : [abs(VVMC_VehicleSpeed_kph - VVMC_RRWhlSpeedRollAve_kph) >= KVMC_SingleWhlSlipRatioTHR_kph]
    (junction 154) -> (junction 169) [order 2]
    (junction 153) -> (junction 152) [order 2]
    (junction 150) -> (junction 155) : {VVMC_SingleWhlSlipRatioCtrl_flg = TRUE}
    (junction 152) -> (junction 169)
    (junction 169) -> (junction 157)
    (junction 157) -> (junction 163) [order 1] : [(VINP_LFRawWhlSpeedV_flg == TRUE &&...
        |   VINP_RFRawWhlSpeedV_flg == TRUE) ||...
        |  (VINP_LRRawWhlSpeedV_flg == TRUE &&...
        |   VINP_RRRawWhlSpeedV_flg == TRUE)]
    (junction 157) -> (junction 167) [order 2] : {VVMC_SingleWhlSlipRatioCtrl_flg = FALSE}
    (junction 163) -> (junction 165) : {VVMC_SingleWhlSlipRatioCtrl_flg = TRUE}
  data: VVMC_VehicleSpeed_kph input single; VVMC_LFWhlSpeedRollAve_kph input single; VVMC_RFWhlSpeedRollAve_kph input single; VVMC_LRWhlSpeedRollAve_kph input single; VVMC_RRWhlSpeedRollAve_kph input single; VINP_LFRawWhlSpeedV_flg input boolean; VINP_RFRawWhlSpeedV_flg input boolean; VINP_LRRawWhlSpeedV_flg input boolean; VINP_RRRawWhlSpeedV_flg input boolean; KVMC_SingleWhlSlipRatioTHR_kph input single; TRUE input boolean; VVMC_SingleWhlSlipRatioCtrl_flg output boolean; FALSE input boolean

== stateflow chart vmc/VMC/VMC/SafetyControl/VehSpdRollingAverage/RollingAverage ==
  state LatAccelRollingAverage
    (default) -> (junction 2) : {VVMC_RollAveCount_enum = ONE_INT}
    LatAccelRollingAverage -> (junction 2)
    (junction 2) -> (junction 3) : {VVMC_VehSpdRollAveRaw_kph = ZERO_FLOAT}
    (junction 3) -> (junction 100) [order 1] : [VVMC_RollAveCount_enum < KVMC_VehSpdRollAveLevel_enum]
    (junction 3) -> (junction 37) [order 2]
    (junction 100) -> (junction 5) : {% Memory
        |  VVMC_Memory_raw32[VVMC_RollAveCount_enum] = VVMC_VehicleSpeedAftLim_kph;
        |
        |  % Memory Shift Counter
        |  VVMC_ShiftCount_enum = ONE_INT}
    (junction 5) -> (junction 7) [order 2]
    (junction 5) -> (junction 6) [order 1] : [VVMC_ShiftCount_enum <= VVMC_RollAveCount_enum]
    (junction 7) -> (junction 8) : {% Rolling Average
        |  VVMC_VehSpdRollAveRaw_kph = VVMC_VehSpdRollAveRaw_kph / VVMC_RollAveCount_enum;
        |
        |  % Rolling Average Counter
        |  VVMC_RollAveCount_enum++}
    (junction 35) -> (junction 5) : {VVMC_ShiftCount_enum++}
    (junction 6) -> (junction 36) : {% Rolling Average Sum
        |  VVMC_VehSpdRollAveRaw_kph = VVMC_VehSpdRollAveRaw_kph + VVMC_Memory_raw32[VVMC_ShiftCount_enum];
        |  }
    (junction 36) -> (junction 35)
    (junction 37) -> (junction 76) [order 1] : [VVMC_RollAveCount_enum == KVMC_VehSpdRollAveLevel_enum]
    (junction 76) -> (junction 47)
    (junction 37) -> (junction 60) [order 2]
    (junction 78) -> (junction 76)
    (junction 47) -> (junction 30) : {% Memory
        |  VVMC_Memory_raw32[VVMC_RollAveCount_enum] = VVMC_VehicleSpeedAftLim_kph;
        |
        |  % Memory Shift Counter
        |  VVMC_ShiftCount_enum = ONE_INT;
        | }
    (junction 60) -> (junction 62) [order 1] : [VVMC_RollAveCount_enum > KVMC_VehSpdRollAveLevel_enum]
    (junction 60) -> (junction 39) [order 2]
    (junction 62) -> (junction 66) : {VVMC_MemoryShiftCount_enum = ONE_INT}
    (junction 30) -> (junction 48) [order 2]
    (junction 30) -> (junction 22) [order 1] : [VVMC_ShiftCount_enum <= VVMC_RollAveCount_enum]
    (junction 48) -> (junction 45) : {% Rolling Average
        |  VVMC_VehSpdRollAveRaw_kph = VVMC_VehSpdRollAveRaw_kph / VVMC_RollAveCount_enum;
        |
        |  % Memory Shift Counter
        |  VVMC_ShiftCount_enum = ONE_INT}
    (junction 14) -> (junction 30) : {VVMC_ShiftCount_enum++}
    (junction 22) -> (junction 25) : {% Rolling Average Sum
        |  VVMC_VehSpdRollAveRaw_kph = VVMC_VehSpdRollAveRaw_kph + VVMC_Memory_raw32[VVMC_ShiftCount_enum]}
    (junction 66) -> (junction 82) [order 2]
    (junction 66) -> (junction 69) [order 1] : [VVMC_MemoryShiftCount_enum < VVMC_RollAveCount_enum]
    (junction 82) -> (junction 80) : {VVMC_RollAveCount_enum = KVMC_VehSpdRollAveLevel_enum}
    (junction 73) -> (junction 66) : {VVMC_MemoryShiftCount_enum++}
    (junction 69) -> (junction 71) : {VVMC_Memory_raw32[VVMC_MemoryShiftCount_enum] =...
        |  VVMC_Memory_raw32[VVMC_RollAveCount_enum - KVMC_VehSpdRollAveLevel_enum + VVMC_MemoryShiftCount_enum]}
    (junction 25) -> (junction 14)
    (junction 71) -> (junction 73)
    (junction 80) -> (junction 78)
    (junction 45) -> (junction 39) [order 2]
    (junction 45) -> (junction 15) [order 1] : [VVMC_ShiftCount_enum < VVMC_RollAveCount_enum]
    (junction 41) -> (junction 45) : { VVMC_ShiftCount_enum++}
    (junction 15) -> (junction 38) : {% Gy Memory Shift
        |  VVMC_Memory_raw32[VVMC_ShiftCount_enum] = VVMC_Memory_raw32[VVMC_ShiftCount_enum + ONE_INT]}
    (junction 38) -> (junction 41)
  data: KVMC_VehSpdRollAveLevel_enum input uint8; VVMC_ShiftCount_enum local uint8; VVMC_RollAveCount_enum local uint8; VVMC_Memory_raw32 local single size=256; ZERO_FLOAT input single; ONE_INT input uint8; VVMC_VehicleSpeedAftLim_kph input single; VVMC_MemoryShiftCount_enum local uint8; VVMC_VehSpdRollAveRaw_kph output single

== stateflow chart vmc/VMC/VMC/SafetyControl/WheelSpeedRollingAverage/RollingAverage ==
  state LatAccelRollingAverage
    (default) -> (junction 2) : {VVMC_RollAveCount_enum = ONE_INT}
    LatAccelRollingAverage -> (junction 2)
    (junction 2) -> (junction 3) : {VVMC_LFWhlSpeedRollAveRaw_kph = ZERO_FLOAT}
    (junction 3) -> (junction 100) [order 1] : [VVMC_RollAveCount_enum < KVMC_WhlSpdRollAveLevel_enum]
    (junction 3) -> (junction 37) [order 2]
    (junction 100) -> (junction 5) : {% Memory
        |  VVMC_Memory_raw32[VVMC_RollAveCount_enum] = VINP_LFRawWhlSpeed_kph;
        |
        |  % Memory Shift Counter
        |  VVMC_ShiftCount_enum = ONE_INT}
    (junction 5) -> (junction 7) [order 2]
    (junction 5) -> (junction 6) [order 1] : [VVMC_ShiftCount_enum <= VVMC_RollAveCount_enum]
    (junction 7) -> (junction 8) : {% Rolling Average
        |  VVMC_LFWhlSpeedRollAveRaw_kph = VVMC_LFWhlSpeedRollAveRaw_kph / VVMC_RollAveCount_enum;
        |
        |  % Rolling Average Counter
        |  VVMC_RollAveCount_enum++}
    (junction 35) -> (junction 5) : {VVMC_ShiftCount_enum++}
    (junction 6) -> (junction 36) : {% Rolling Average Sum
        |  VVMC_LFWhlSpeedRollAveRaw_kph = VVMC_LFWhlSpeedRollAveRaw_kph + VVMC_Memory_raw32[VVMC_ShiftCount_enum];
        |  }
    (junction 36) -> (junction 35)
    (junction 37) -> (junction 76) [order 1] : [VVMC_RollAveCount_enum == KVMC_WhlSpdRollAveLevel_enum]
    (junction 76) -> (junction 47)
    (junction 37) -> (junction 60) [order 2]
    (junction 78) -> (junction 76)
    (junction 47) -> (junction 30) : {% Memory
        |  VVMC_Memory_raw32[VVMC_RollAveCount_enum] = VINP_LFRawWhlSpeed_kph;
        |
        |  % Memory Shift Counter
        |  VVMC_ShiftCount_enum = ONE_INT;
        | }
    (junction 60) -> (junction 62) [order 1] : [VVMC_RollAveCount_enum > KVMC_WhlSpdRollAveLevel_enum]
    (junction 60) -> (junction 39) [order 2]
    (junction 62) -> (junction 66) : {VVMC_MemoryShiftCount_enum = ONE_INT}
    (junction 30) -> (junction 48) [order 2]
    (junction 30) -> (junction 22) [order 1] : [VVMC_ShiftCount_enum <= VVMC_RollAveCount_enum]
    (junction 48) -> (junction 45) : {% Rolling Average
        |  VVMC_LFWhlSpeedRollAveRaw_kph = VVMC_LFWhlSpeedRollAveRaw_kph / VVMC_RollAveCount_enum;
        |
        |  % Memory Shift Counter
        |  VVMC_ShiftCount_enum = ONE_INT}
    (junction 14) -> (junction 30) : {VVMC_ShiftCount_enum++}
    (junction 22) -> (junction 25) : {% Rolling Average Sum
        |  VVMC_LFWhlSpeedRollAveRaw_kph = VVMC_LFWhlSpeedRollAveRaw_kph + VVMC_Memory_raw32[VVMC_ShiftCount_enum]}
    (junction 66) -> (junction 82) [order 2]
    (junction 66) -> (junction 69) [order 1] : [VVMC_MemoryShiftCount_enum < VVMC_RollAveCount_enum]
    (junction 82) -> (junction 80) : {VVMC_RollAveCount_enum = KVMC_WhlSpdRollAveLevel_enum}
    (junction 73) -> (junction 66) : {VVMC_MemoryShiftCount_enum++}
    (junction 69) -> (junction 71) : {VVMC_Memory_raw32[VVMC_MemoryShiftCount_enum] =...
        |  VVMC_Memory_raw32[VVMC_RollAveCount_enum - KVMC_WhlSpdRollAveLevel_enum + VVMC_MemoryShiftCount_enum]}
    (junction 25) -> (junction 14)
    (junction 71) -> (junction 73)
    (junction 80) -> (junction 78)
    (junction 45) -> (junction 39) [order 2]
    (junction 45) -> (junction 15) [order 1] : [VVMC_ShiftCount_enum < VVMC_RollAveCount_enum]
    (junction 41) -> (junction 45) : { VVMC_ShiftCount_enum++}
    (junction 15) -> (junction 38) : {% Gy Memory Shift
        |  VVMC_Memory_raw32[VVMC_ShiftCount_enum] = VVMC_Memory_raw32[VVMC_ShiftCount_enum + ONE_INT]}
    (junction 38) -> (junction 41)
  data: KVMC_WhlSpdRollAveLevel_enum input uint8; VVMC_ShiftCount_enum local uint8; VVMC_RollAveCount_enum local uint8; VVMC_Memory_raw32 local single size=256; ZERO_FLOAT input single; ONE_INT input uint8; VINP_LFRawWhlSpeed_kph input single; VVMC_MemoryShiftCount_enum local uint8; VVMC_LFWhlSpeedRollAveRaw_kph output single
